simulink subsystem "Volume_flow"  (R2025b)
settings: Solver=VariableStepAuto  StartTime=0.0  StopTime=10.0  RelTol=1e-3
model mask{InitialCondition=100, Max_cap=10, Diameter=24.5, K=7.77*1e-5, Height=1, A=0.0117, B=0.1252}
  mask prompts: InitialCondition "Initial level:"; Max_cap "Max capacity"; A "Valve coeff A:"; B "Valve coeff B:"
settings Model: Creator=Soere  LastModifiedBy=klump

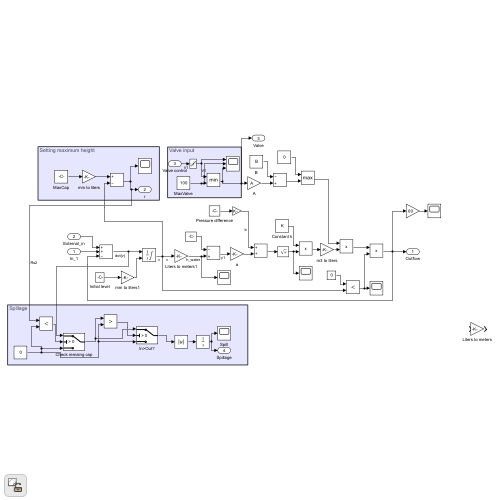
[thumbnail: Simulink's stored preview of the top-level diagram]
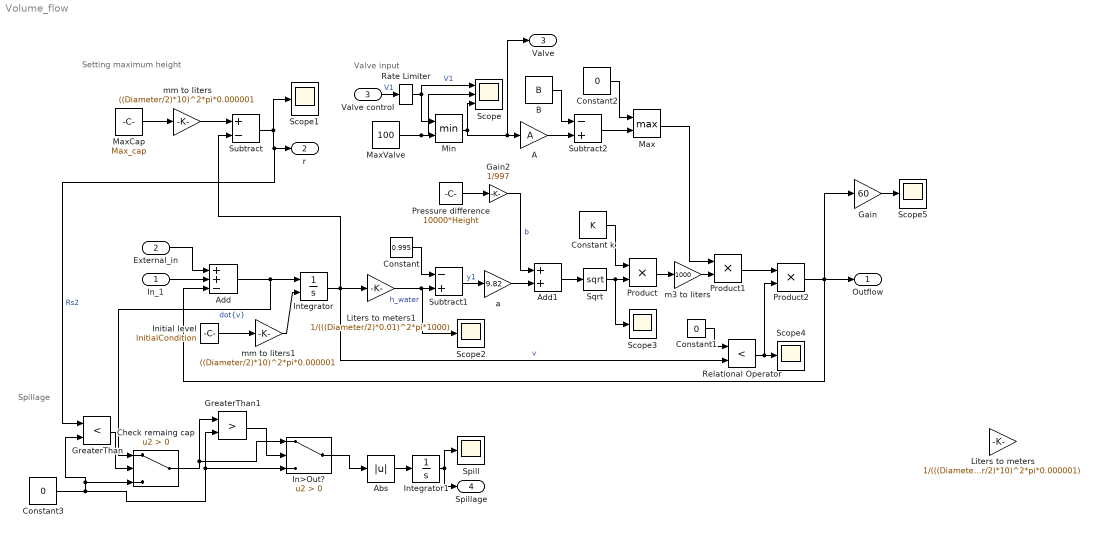
== system Volume_flow ==
  note: Spillage
  note: Setting maximum height
  note: Valve input
  In_1 : Inport
  External_in : Inport  Port=2
  Valve control : Inport  Port=3  OutMin=0  OutMax=100
  A : Gain  Gain=A
  Abs : Abs  SaturateOnIntegerOverflow=off
  Add : Sum  Inputs=++-
  Add1 : Sum
  B : Constant  Value=B
  Check remaing cap : Switch  Criteria=u2 > Threshold  SaturateOnIntegerOverflow=off  InputSameDT=off
  Constant : Constant  Value=0.995
  Constant k : Constant  Value=K
  Constant1 : Constant  Value=0
  Constant2 : Constant  Value=0
  Constant3 : Constant  Value=0
  Gain : Gain  Gain=60
  Gain2 : Gain  Gain=1/997
  GreaterThan : RelationalOperator  Operator=<  OutDataTypeStr=boolean  RndMeth=Simplest  InputSameDT=off
  GreaterThan1 : RelationalOperator  Operator=>  OutDataTypeStr=boolean  RndMeth=Simplest  InputSameDT=off
  In>Out? : Switch  Criteria=u2 > Threshold  SaturateOnIntegerOverflow=off  InputSameDT=off
  Initial level : Constant  Value=InitialCondition
  Integrator : Integrator  InitialConditionSource=external  InitialCondition=100  LimitOutput=on  UpperSaturationLimit=Max_cap  LowerSaturationLimit=0
  Integrator1 : Integrator
  Liters to meters : Gain  Gain=1/(((Diameter/2)*10)^2*pi*0.000001)
  Liters to meters1 : Gain  Gain=1/(((Diameter/2)*0.01)^2*pi*1000)
  Max : MinMax  Function=max  Inputs=2
  MaxCap : Constant  Value=Max_cap
  MaxValve : Constant  Value=100  SampleTime=-1
  Min : MinMax  Inputs=2
  Pressure difference : Constant  Value=10000*Height
  Product : Product
  Product1 : Product
  Product2 : Product
  Rate Limiter : RateLimiter  RisingSlewLimit=11.11  FallingSlewLimit=-11.11  SampleTimeMode=inherited
  Relational Operator : RelationalOperator  Operator=<  OutDataTypeStr=boolean  RndMeth=Simplest  InputSameDT=off
  Scope : Scope  NumInputPorts=3
      settings: ActiveDisplayYMinimum=-16.555361778066185  ActiveDisplayYMaximum=118.63213822193381  DataLoggingVariableName=ScopeData44
  Scope{1..5} (5 alike) : Scope
      Scope1 settings: ActiveDisplayYMinimum=-16.555361778066185  ActiveDisplayYMaximum=118.63213822193381  DataLoggingVariableName=ScopeData54
      Scope2 settings: ActiveDisplayYMinimum=-0.0735491371491241  ActiveDisplayYMaximum=0.66194223434211708  DataLoggingVariableName=ScopeData55
      Scope3 settings: ActiveDisplayYMinimum=-1  ActiveDisplayYMaximum=1  DataLoggingVariableName=ScopeData56
      Scope4 settings: ActiveDisplayYMinimum=-1  ActiveDisplayYMaximum=1  DataLoggingVariableName=ScopeData57
      Scope5 settings: ActiveDisplayYMinimum=-1.2246856264436343  ActiveDisplayYMaximum=11.02217063799271  DataLoggingVariableName=ScopeData58
  Spill : Scope
      settings: ActiveDisplayYMinimum=-0.46221271341368758  ActiveDisplayYMaximum=4.1599144207231893  DataLoggingVariableName=ScopeData59
  Sqrt : Sqrt
  Subtract : Sum  Inputs=+-
  Subtract1 : Sum  Inputs=-+
  Subtract2 : Sum  Inputs=-+
  a : Gain  Gain=9.82
  m3 to liters : Gain  Gain=1000
  mm to liters : Gain  Gain=((Diameter/2)*10)^2*pi*0.000001
  mm to liters1 : Gain  Gain=((Diameter/2)*10)^2*pi*0.000001
  Outflow : Outport
  r : Outport  Port=2
  Valve : Outport  Port=3
  Spillage : Outport  Port=4
  wires:
  Relational Operator/1 -> Scope4/1, Product2/2
  Constant1/1 -> Relational Operator/1
  Product2/1 -> Add/3, Outflow/1, Gain/1
  Product1/1 -> Product2/1
  mm to liters1/1 -> Integrator/2
  B/1 -> Subtract2/1
  Subtract2/1 -> Max/2
  Constant2/1 -> Max/1
  A/1 -> Subtract2/2
  Constant k/1 -> Product/1
  Sqrt/1 -> Scope3/1, Product/2
  Add1/1 -> Sqrt/1
  Gain2/1 -> Add1/1  "b"
  Pressure difference/1 -> Gain2/1
  a/1 -> Add1/2
  Subtract1/1 -> a/1  "y1"
  Constant/1 -> Subtract1/1
  Liters to meters1/1 -> Subtract1/2, Scope2/1  "h_water"
  Initial level/1 -> mm to liters1/1
  mm to liters/1 -> Subtract/1
  MaxCap/1 -> mm to liters/1
  MaxValve/1 -> Scope/2, Min/2
  Min/1 -> A/1, Valve/1, Scope/3
  Add/1 -> Integrator/1, Check remaing cap/1  "dot{v}"
  Integrator/1 -> Relational Operator/2, Liters to meters1/1, Subtract/2  "v"
  Max/1 -> Product1/1
  Product/1 -> m3 to liters/1
  m3 to liters/1 -> Product1/2
  Valve control/1 -> Rate Limiter/1  "V1"
  Rate Limiter/1 -> Scope/1, Min/1  "V1"
  Gain/1 -> Scope5/1
  In_1/1 -> Add/2
  External_in/1 -> Add/1
  Subtract/1 -> Scope1/1, GreaterThan/1, r/1  "Rs2"
  Integrator1/1 -> Spillage/1, Spill/1
  Constant3/1 -> GreaterThan/2, Check remaing cap/3, GreaterThan1/2, In>Out?/3
  Abs/1 -> Integrator1/1
  GreaterThan/1 -> Check remaing cap/2
  Check remaing cap/1 -> GreaterThan1/1, In>Out?/1
  GreaterThan1/1 -> In>Out?/2
  In>Out?/1 -> Abs/1
